simulink model "send_a429_r2020b"  (R2020b)
settings: Solver=VariableStepAuto  StartTime=0.0  StopTime=10.0  RelTol=1e-3
PreLoadFcn:
  | ds = Simulink.SimulationData.Dataset();
  | ds = ds.addElement(timeseries(uint8((1:11)' + (1:4)),       (0:10)', 'Name', 'AnA429SamplingMessage'),   'Name', 'AnA429SamplingMessage');
  | ds = ds.addElement(timeseries(uint8((250:-1:240)' + (1:4)), (0:10)', 'Name', 'AnA429QueuingMessage'),    'Name', 'AnA429QueuingMessage');
libraries: lib_ed247 x2
settings Model: EnablePacing=on  Creator=odufour  LastModifiedBy=odufour
settings DataIOCC: ExternalInput=ds  LoadExternalInput=on

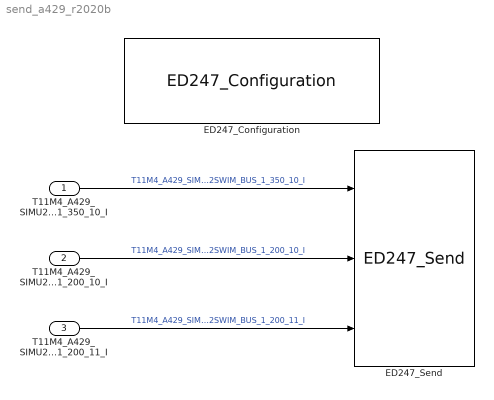
== system send_a429_r2020b ==
  T11M4_A429_SIMU2SWIM_BUS_1_350_10_I : Inport  OutDataTypeStr=uint8  PortDimensions=4  SampleTime=0.1
  T11M4_A429_SIMU2SWIM_BUS_1_200_10_I : Inport  Port=2  OutDataTypeStr=uint8  PortDimensions=4  SampleTime=0.1
  T11M4_A429_SIMU2SWIM_BUS_1_200_11_I : Inport  Port=3  OutDataTypeStr=uint8  PortDimensions=4  SampleTime=0.1
  ED247_Configuration : lib_ed247/ED247_Configuration  configurationFilename='ecic_func_exchange_a429_uc_main_simple.xml'  enableLog=off  logFilename=''
      settings: SourceProductName=Airbus ED247
  ED247_Send : lib_ed247/ED247_Send  Parameter1=0
      settings: SourceProductName=Airbus ED247
  wires:
  T11M4_A429_SIMU2SWIM_BUS_1_350_10_I/1 -> ED247_Send/1  "T11M4_A429_SIMU2SWIM_BUS_1_350_10_I"
  T11M4_A429_SIMU2SWIM_BUS_1_200_10_I/1 -> ED247_Send/2  "T11M4_A429_SIMU2SWIM_BUS_1_200_10_I"
  T11M4_A429_SIMU2SWIM_BUS_1_200_11_I/1 -> ED247_Send/3  "T11M4_A429_SIMU2SWIM_BUS_1_200_11_I"
